simulink model "OFDM"  (R2023a)
settings: Solver=VariableStepAuto  StartTime=0.0  StopTime=3  RelTol=1e-3
libraries: commofdm x2, commchan3 x1, commrandsrc3 x1, commdigbbndpm3 x1
settings Model: Creator=marta  LastModifiedBy=marta

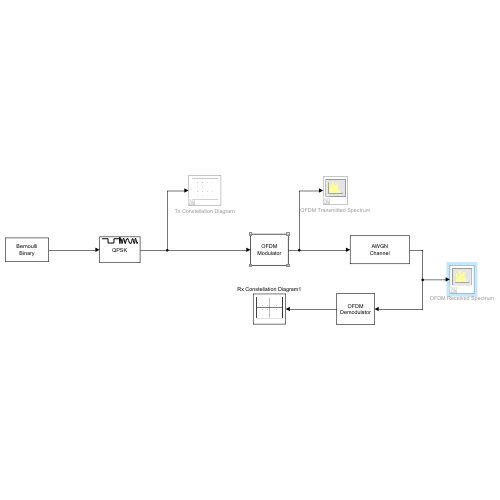
[thumbnail: Simulink's stored preview of the top-level diagram]
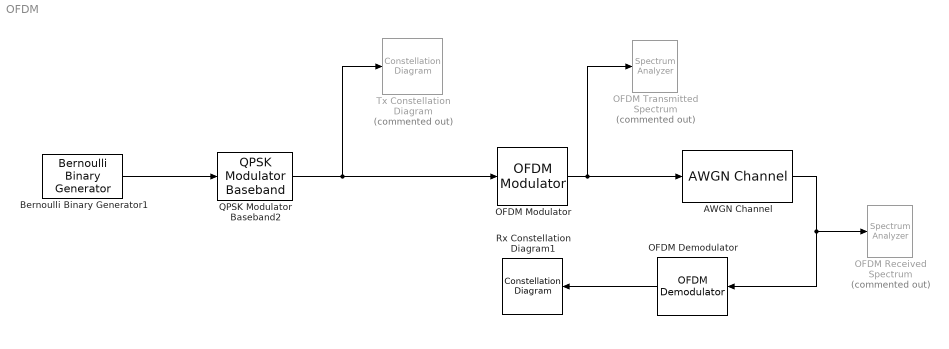
== system OFDM ==
  AWGN Channel : commchan3/AWGN Channel  LegacyMode=off  NoiseMethod="Signal to noise ratio  (SNR)"  noiseMode="Signal to noise ratio  (SNR)"  EbNo=10  EsNo=10  SNR=20  BitsPerSymbol=1  SignalPower=1  SamplesPerSymbol=1  SymbolPeriod=1  VarianceSource=Parameter  Variance=1  RandomStream=Global stream  Seed=67  SimulateUsing=Interpreted execution
  Bernoulli Binary Generator1 : commrandsrc3/Bernoulli Binary Generator  ProbabilityOfZero=0.5  SeedSource=Auto  Seed=0  SampleTime=1e-6  SamplesPerFrame=106  OutputDataType=double  SimulateUsing=Interpreted execution
  OFDM Demodulator : commofdm/OFDM Demodulator  StatePerturbationForJacobian=1.0e-05  FFTLength=64  NumGuardBandCarriers=[6; 5]  RemoveDCCarrier=off  PilotOutputPort=off  PilotCarrierIndices=[12; 26; 40; 54]  CyclicPrefixLength=16  OversamplingFactor=1  NumSymbols=1  NumReceiveAntennas=1  SimulateUsing=Interpreted execution
  OFDM Modulator : commofdm/OFDM Modulator  StatePerturbationForJacobian=1.0e-05  FFTLength=64  NumGuardBandCarriers=[6; 5]  InsertDCNull=off  PilotInputPort=off  PilotCarrierIndices=[12; 26; 40; 54]  CyclicPrefixLength=16  Windowing=off  WindowLength=1  OversamplingFactor=1  NumSymbols=1  NumTransmitAntennas=1  SimulateUsing=Interpreted execution
  OFDM Received Spectrum : SpectrumAnalyzer  Commented=on  WindowPosition=[302.000000,44.000000,800.000000,500.000000,]  ScopeFrameLocation=window  YLimits=[-24.74219953,-12.14375095]  ColorLimits=[-80 20]
  OFDM Transmitted Spectrum : SpectrumAnalyzer  Commented=on  WindowPosition=[284.000000,111.000000,800.000000,500.000000,]  ScopeFrameLocation=window  YLimits=[-42.10975515,-12.34758527]  ColorLimits=[-80 20]
  QPSK Modulator Baseband2 : commdigbbndpm3/QPSK Modulator Baseband  InType=Bit  Enc=Gray  Ph=pi/4  outDtype=double  outWordLen=16  outUDDataType=sfix(16)  outFracLenMode=Best precision  outFracLen=15  outDataTypeStr=double  outLastDataTypeStr=double
  Rx Constellation Diagram1 : ConstellationDiagram  WindowPosition=[450.000000,46.000000,600.000000,600.000000,]  ScopeFrameLocation=window
  Tx Constellation Diagram : ConstellationDiagram  Commented=on  WindowPosition=[450.000000,46.000000,600.000000,600.000000,]  ScopeFrameLocation=window
  wires:
  Bernoulli Binary Generator1/1 -> QPSK Modulator Baseband2/1
  QPSK Modulator Baseband2/1 -> OFDM Modulator/1, Tx Constellation Diagram/1
  OFDM Modulator/1 -> OFDM Transmitted Spectrum/1, AWGN Channel/1
  AWGN Channel/1 -> OFDM Received Spectrum/1, OFDM Demodulator/1
  OFDM Demodulator/1 -> Rx Constellation Diagram1/1
